simulink model "IM_Control_Sim_Current_Flux"  (R2024b)
settings: Solver=VariableStepAuto  StartTime=0.0  StopTime=200  RelTol=1e-3
InitFcn:
  | IM_parameters_init;
undefined symbols (not defined in the file): ctrl, im, Lm, Lr, Ls, p, Rr
libraries: simulink x2
settings Model: Creator=matth  LastModifiedBy=overflow

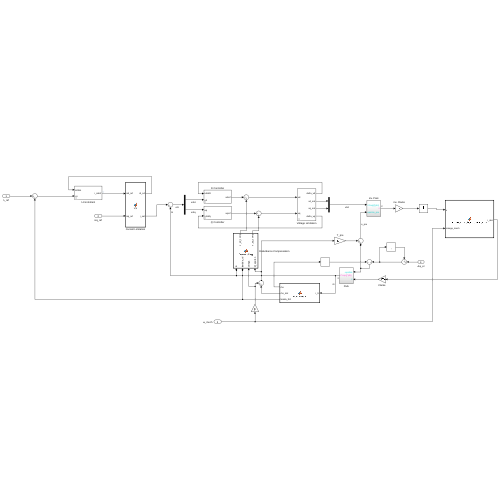
[thumbnail: Simulink's stored preview of the top-level diagram]
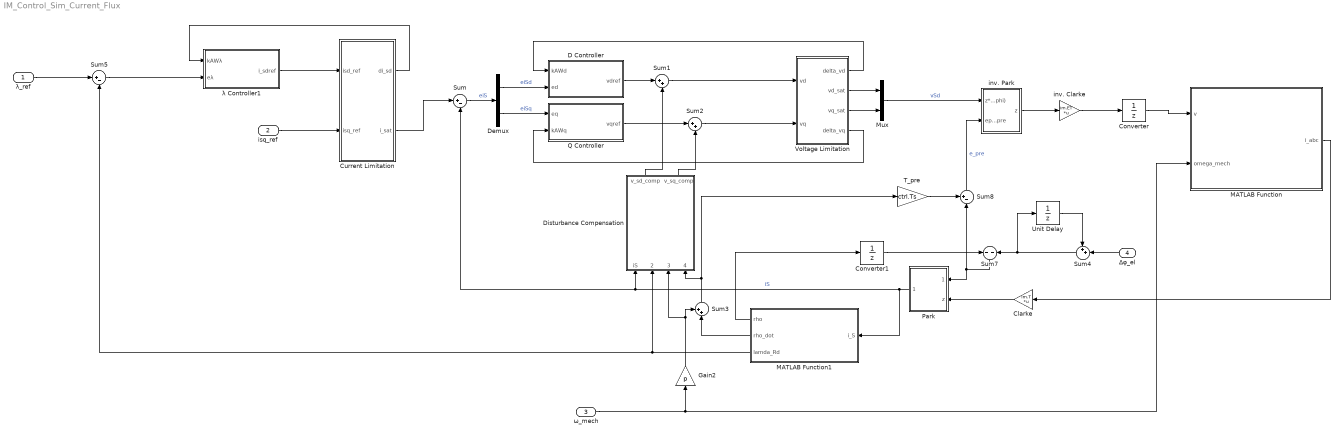
== system IM_Control_Sim_Current_Flux ==
  λ_ref : Inport
  isq_ref : Inport  Port=2
  ω_mech : Inport  Port=3
  Δφ_el : Inport  Port=4
  Clarke : Gain  Gain=im.T  Multiplication=Matrix(K*u)
  Converter : UnitDelay  SampleTime=-1  HasFrameUpgradeWarning=on
  Converter1 : UnitDelay  SampleTime=-1  HasFrameUpgradeWarning=on
  Current Limitation : MATLAB Function  TreatAsAtomicUnit=on
  D Controller : Subsystem  mask{Ts=ctrl.Ts, ctrl=ctrl.i}
      mask prompts: Ts "Sampling Time"; ctrl "Controller Struct"
  Demux : Demux  Outputs=2
  Disturbance Compensation : MATLAB Function  TreatAsAtomicUnit=on
  Gain2 : Gain  Gain=p
  MATLAB Function : MATLAB Function  TreatAsAtomicUnit=on
  MATLAB Function1 : MATLAB Function  TreatAsAtomicUnit=on
  Mux : Mux  Inputs=2
  Park : Subsystem
  Q Controller : Subsystem  mask{Ts=ctrl.Ts, ctrl=ctrl.i}
      mask prompts: Ts "Sampling Time"; ctrl "Controller Struct"
  Sum : Sum  Inputs=|+-
  Sum1 : Sum  Inputs=|++  OutDataTypeStr=double  AccumDataTypeStr=double
  Sum2 : Sum  Inputs=|++  OutDataTypeStr=double  AccumDataTypeStr=double
  Sum3 : Sum  Inputs=++|
  Sum4 : Sum  Inputs=++|
  Sum5 : Sum  Inputs=|+-
  Sum7 : Sum  Inputs=-|-
  Sum8 : Sum  Inputs=+-|
  T_pre : Gain  Gain=ctrl.Ts  SaturateOnIntegerOverflow=on  OutDataTypeStr=Inherit: Same as input  ParamDataTypeStr=Inherit: Same as input
  Unit Delay : UnitDelay  SampleTime=-1  HasFrameUpgradeWarning=on
  Voltage Limitation : Subsystem  mask{Vmax=im.vDC}
      mask prompts: Vmax "Max Voltage"
  inv. Clarke : Gain  Gain=im.ET  Multiplication=Matrix(K*u)
  inv. Park : Subsystem
  λ Controller1 : Subsystem  mask{Ts=ctrl.Ts, ctrl=ctrl.w}
      mask prompts: Ts "Sampling Time"; ctrl "Controller Struct"
  wires:
  Q Controller/1(vqref) -> Sum2/1
  Sum2/1 -> Voltage Limitation/2("vq ")
  Sum1/1 -> Voltage Limitation/1(vd)
  D Controller/1(vdref) -> Sum1/1
  Voltage Limitation/3(vq_sat) -> Mux/2
  MATLAB Function/1(i_abc) -> Clarke/1
  Mux/1 -> inv. Park/1(z*exp(j*phi))  "vSd"
  Voltage Limitation/1(delta_vd) -> D Controller/1(kAWd)
  Sum/1 -> Demux/1  "eiS"
  Demux/1 -> D Controller/2(ed)  "eiSd"
  Clarke/1 -> Park/2(z)
  inv. Park/1(z) -> inv. Clarke/1
  Demux/2 -> Q Controller/1(eq)  "eiSq"
  Park/1(z*exp(j*phi)) -> MATLAB Function1/1(i_S), Disturbance Compensation/1(iS), Sum/2  "iS"
  Voltage Limitation/4(delta_vq) -> Q Controller/2(kAWq)
  Voltage Limitation/2(vd_sat) -> Mux/1
  Converter/1 -> MATLAB Function/1(v)
  MATLAB Function1/3(lamda_Rd) -> Disturbance Compensation/2(lambda_rd), Sum5/2
  Sum3/1 -> Disturbance Compensation/4(dt_epsilon), T_pre/1
  Current Limitation/2(i_sat) -> Sum/1
  MATLAB Function1/2(rho_dot) -> Sum3/2
  Sum7/1 -> Park/1(-epsilon), Sum8/2
  T_pre/1 -> Sum8/1
  MATLAB Function1/1(rho) -> Converter1/1
  Converter1/1 -> Sum7/1
  λ Controller1/1(i_sdref) -> Current Limitation/1(isd_ref)
  Current Limitation/1(di_sd) -> λ Controller1/1(kAWλ)
  Sum5/1 -> λ Controller1/2(eλ)
  λ_ref/1 -> Sum5/1
  inv. Clarke/1 -> Converter/1
  isq_ref/1 -> Current Limitation/2(isq_ref)
  Sum8/1 -> inv. Park/2(epsilon_pre)  "e_pre"
  Disturbance Compensation/1(v_sd_comp) -> Sum1/2
  Disturbance Compensation/2(v_sq_comp) -> Sum2/2
  Gain2/1 -> Sum3/1, Disturbance Compensation/3(omega)
  ω_mech/1 -> Gain2/1, MATLAB Function/2(omega_mech)
  Δφ_el/1 -> Sum4/2
  Sum4/1 -> Unit Delay/1, Sum7/2
  Unit Delay/1 -> Sum4/1

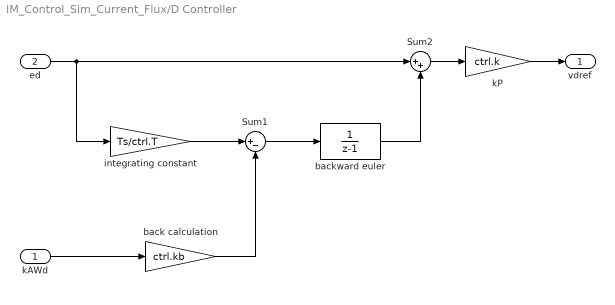
== system IM_Control_Sim_Current_Flux/D Controller ==
  kAWd : Inport
  ed : Inport  Port=2
  Sum1 : Sum  Inputs=|+-
  Sum2 : Sum  Inputs=|++
  back calculation : Gain  Gain=ctrl.kb
  backward euler : DiscreteTransferFcn  Denominator=[1 -1]
  integrating constant : Gain  Gain=Ts/ctrl.T
  kP : Gain  Gain=ctrl.k
  vdref : Outport
  wires:
  Sum1/1 -> backward euler/1
  integrating constant/1 -> Sum1/1
  back calculation/1 -> Sum1/2
  ed/1 -> integrating constant/1, Sum2/1
  Sum2/1 -> kP/1
  kP/1 -> vdref/1
  backward euler/1 -> Sum2/2
  kAWd/1 -> back calculation/1

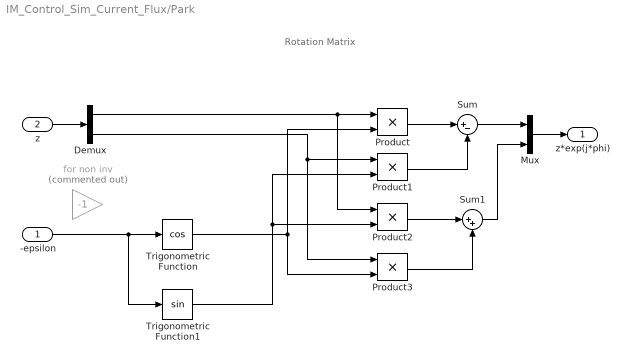
== system IM_Control_Sim_Current_Flux/Park ==
  note: Rotation Matrix
  -epsilon : Inport
  z : Inport  Port=2
  Demux : Demux  Outputs=2
      settings: DisplayOption=none
  Mux : Mux  Inputs=2
  Product{,1..3} (4 alike) : Product  SaturateOnIntegerOverflow=on  OutDataTypeStr=Inherit: Same as first input
  Sum : Sum  Inputs=|+-  SaturateOnIntegerOverflow=on
  Sum1 : Sum  Inputs=|++  SaturateOnIntegerOverflow=on
  Trigonometric Function : Trigonometry  Operator=cos
  Trigonometric Function1 : Trigonometry
  for non inv : Gain  Commented=on  Gain=-1
  z*exp(j*phi) : Outport  PortDimensions=2  VectorParamsAs1DForOutWhenUnconnected=off
  wires:
  Mux/1 -> z*exp(j*phi)/1
  Sum1/1 -> Mux/2
  Sum/1 -> Mux/1
  Product3/1 -> Sum1/2
  Product2/1 -> Sum1/1
  Product1/1 -> Sum/2
  Product/1 -> Sum/1
  Trigonometric Function1/1 -> Product2/2, Product1/2
  Trigonometric Function/1 -> Product3/2, Product/2
  Demux/2 -> Product3/1, Product1/1
  Demux/1 -> Product2/1, Product/1
  z/1 -> Demux/1
  -epsilon/1 -> Trigonometric Function1/1, Trigonometric Function/1

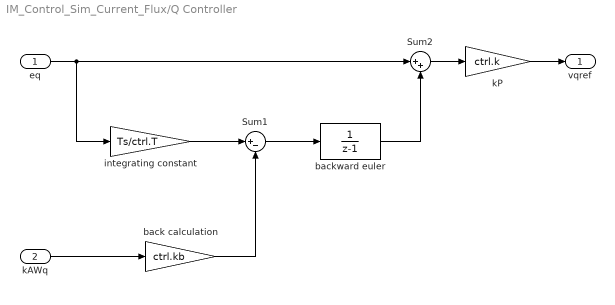
== system IM_Control_Sim_Current_Flux/Q Controller ==
  eq : Inport
  kAWq : Inport  Port=2
  Sum1 : Sum  Inputs=|+-
  Sum2 : Sum  Inputs=|++
  back calculation : Gain  Gain=ctrl.kb
  backward euler : DiscreteTransferFcn  Denominator=[1 -1]
  integrating constant : Gain  Gain=Ts/ctrl.T
  kP : Gain  Gain=ctrl.k
  vqref : Outport
  wires:
  Sum1/1 -> backward euler/1
  integrating constant/1 -> Sum1/1
  back calculation/1 -> Sum1/2
  eq/1 -> integrating constant/1, Sum2/1
  Sum2/1 -> kP/1
  kP/1 -> vqref/1
  backward euler/1 -> Sum2/2
  kAWq/1 -> back calculation/1

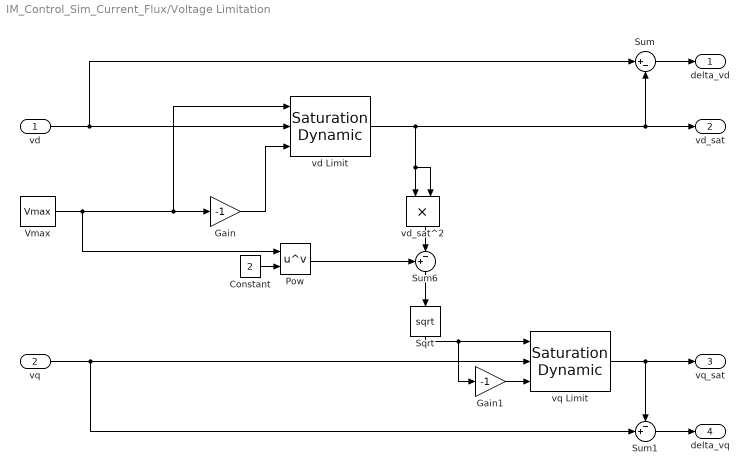
== system IM_Control_Sim_Current_Flux/Voltage Limitation ==
  vd : Inport
  "vq " : Inport  Port=2
  Constant : Constant  Value=2
  Gain : Gain  Gain=-1
  Gain1 : Gain  Gain=-1
  Pow : Math  Operator=pow  RndMeth=Zero
  Sqrt : Sqrt
  Sum : Sum  Inputs=|+-
  Sum1 : Sum  Inputs=-+|
  Sum6 : Sum  Inputs=+-|
  Vmax : Constant  Value=Vmax
  vd Limit : simulink/Discontinuities/Saturation Dynamic  OutMin=[]  OutMax=[]  OutDataTypeStr=Inherit: Same as second input  OutDataType=fixdt(1, 16)  OutScaling=2^-10  DoSatur=off
  vd_sat^2 : Product
  vq Limit : simulink/Discontinuities/Saturation Dynamic  OutMin=[]  OutMax=[]  OutDataTypeStr=Inherit: Same as second input  OutDataType=fixdt(1, 16)  OutScaling=2^-10  DoSatur=off
  delta_vd : Outport  VectorParamsAs1DForOutWhenUnconnected=off
  vd_sat : Outport  Port=2  VectorParamsAs1DForOutWhenUnconnected=off
  vq_sat : Outport  Port=3  VectorParamsAs1DForOutWhenUnconnected=off
  delta_vq : Outport  Port=4  VectorParamsAs1DForOutWhenUnconnected=off
  wires:
  Gain/1 -> vd Limit/3
  vd Limit/1 -> Sum/2, vd_sat/1, vd_sat^2/2, vd_sat^2/1
  Sqrt/1 -> Gain1/1, vq Limit/1
  vq Limit/1 -> Sum1/1, vq_sat/1
  Pow/1 -> Sum6/1
  vd/1 -> Sum/1, vd Limit/2
  Sum6/1 -> Sqrt/1
  "vq "/1 -> vq Limit/2, Sum1/2
  vd_sat^2/1 -> Sum6/2
  Vmax/1 -> Pow/1, Gain/1, vd Limit/1
  Gain1/1 -> vq Limit/3
  Sum/1 -> delta_vd/1
  Sum1/1 -> delta_vq/1
  Constant/1 -> Pow/2

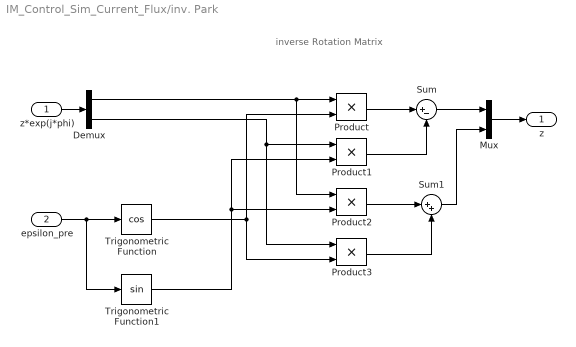
== system IM_Control_Sim_Current_Flux/inv. Park ==
  note: inverse Rotation Matrix
  z*exp(j*phi) : Inport
  epsilon_pre : Inport  Port=2
  Demux : Demux  Outputs=2
      settings: DisplayOption=none
  Mux : Mux  Inputs=2
  Product{,1..3} (4 alike) : Product  SaturateOnIntegerOverflow=on  OutDataTypeStr=Inherit: Same as first input
  Sum : Sum  Inputs=|+-  SaturateOnIntegerOverflow=on
  Sum1 : Sum  Inputs=|++  SaturateOnIntegerOverflow=on
  Trigonometric Function : Trigonometry  Operator=cos
  Trigonometric Function1 : Trigonometry
  z : Outport  PortDimensions=2  VectorParamsAs1DForOutWhenUnconnected=off
  wires:
  z*exp(j*phi)/1 -> Demux/1
  Demux/1 -> Product/1, Product2/1
  epsilon_pre/1 -> Trigonometric Function1/1, Trigonometric Function/1
  Demux/2 -> Product1/1, Product3/1
  Trigonometric Function/1 -> Product/2, Product3/2
  Trigonometric Function1/1 -> Product1/2, Product2/2
  Product/1 -> Sum/1
  Product1/1 -> Sum/2
  Product2/1 -> Sum1/1
  Product3/1 -> Sum1/2
  Sum/1 -> Mux/1
  Sum1/1 -> Mux/2
  Mux/1 -> z/1

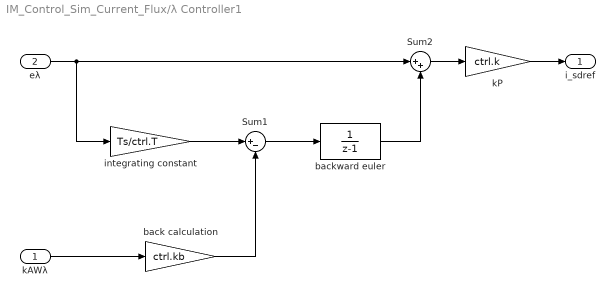
== system IM_Control_Sim_Current_Flux/λ Controller1 ==
  kAWλ : Inport
  eλ : Inport  Port=2
  Sum1 : Sum  Inputs=|+-
  Sum2 : Sum  Inputs=|++
  back calculation : Gain  Gain=ctrl.kb
  backward euler : DiscreteTransferFcn  Denominator=[1 -1]
  integrating constant : Gain  Gain=Ts/ctrl.T
  kP : Gain  Gain=ctrl.k
  i_sdref : Outport
  wires:
  Sum1/1 -> backward euler/1
  integrating constant/1 -> Sum1/1
  back calculation/1 -> Sum1/2
  eλ/1 -> integrating constant/1, Sum2/1
  Sum2/1 -> kP/1
  kP/1 -> i_sdref/1
  backward euler/1 -> Sum2/2
  kAWλ/1 -> back calculation/1

== matlab function IM_Control_Sim_Current_Flux/MATLAB Function1 ==
  data: rho output; rho_dot output; i_S input; lamda_Rd output; par parameter
function [rho, rho_dot, lamda_Rd] = flux_model(i_S, par)

i_sd = i_S(1);
i_sq = i_S(2);

% PARAMETERS
Ts = par.Ts;
p  = par.p;
Jm = par.J;

Rs = par.Rs;
Rr = par.Rr;

Ls = par.Ls;     % LσS
Lr = par.Lr;     % L'σR
Lm  = par.Lm;

Tau_R = Lr/Rr;

persistent rho_k lamda_Rd_k
if isempty(rho_k)
    rho_k = 0;
    lamda_Rd_k = 0.001;
end


lamda_Rd_k = lamda_Rd_k + Ts / Tau_R * (Lm * i_sd - lamda_Rd_k);

lamda_Rd_k = max(lamda_Rd_k, 0.001);


rho_dot = Lm * i_sq / (Tau_R * lamda_Rd_k);

rho_k = rho_k + Ts * rho_dot;

lamda_Rd = lamda_Rd_k;
rho = rho_k;

== matlab function IM_Control_Sim_Current_Flux/Disturbance Compensation ==
  data: iS input; v_sd_comp output; lambda_rd input; omega input; dt_epsilon input; Ls parameter; Lm parameter; Lr parameter; Rr parameter; v_sq_comp output
function [v_sd_comp, v_sq_comp]  = Decoupling(iS, lambda_rd, omega, dt_epsilon, Ls, Lm, Lr, Rr)

i_Sd = iS(1);
i_Sq = iS(2);

% convenience;  (3.15) unter satz
L_sigma=(Ls - Lm^2/Lr); 

% compensation
v_sd_comp = -dt_epsilon*L_sigma*i_Sq - Rr *  Lm/Lr^2 * lambda_rd;  % (3.21)
v_sq_comp =  dt_epsilon*L_sigma*i_Sd + omega * Lm/Lr^2 * lambda_rd; % (3.22)

== matlab function IM_Control_Sim_Current_Flux/MATLAB Function ==
  data: i_abc output; v input; par parameter; omega_mech input
function i_abc  = IM_mech_subsystem_vector(v,par, omega_mech)

va = v(1);
vb = v(2);
vc = v(3);

% PARAMETERS
Ts = par.Ts;
p  = par.p;

Rs = par.Rs;
Rr = par.Rr;

Ls = par.Ls;     
Lr = par.Lr;     
Lm  = par.Lm;


% Persistent states
persistent is_a is_b psir_a psir_b
if isempty(is_a)
    is_a = 0; is_b = 0;
    psir_a = 0; psir_b = 0;
end

% Clarke transform (abc -> alpha-beta), power-invariant
v_alpha = (2/3)*(va - 0.5*vb - 0.5*vc);
v_beta  = (2/3)*((sqrt(3)/2)*(vb - vc));

% Helpful constants
Lsigma = Ls - (Lm^2)/Lr;        % must be > 0
omega_r = p * omega_mech;

% Current and rotor flux vectors
is  = [is_a;  is_b];
psir = [psir_a; psir_b];

Jmat = [0 -1; 1 0];

% Rotor flux derivative: dpsir/dt
dpsir = -(Rr/Lr)*psir + (Rr*Lm/Lr)*is + omega_r*(Jmat*psir);

% Stator current derivative: dis/dt
vs = [v_alpha; v_beta];
dis = (1/Lsigma) * (vs - Rs*is - (Lm/Lr)*dpsir);

% Integrate (Euler)
psir = psir + Ts*dpsir;
is   = is   + Ts*dis;


% Save states back
is_a = is(1); is_b = is(2);
psir_a = psir(1); psir_b = psir(2);


% Inverse Clarke: alpha-beta -> abc currents (with ia+ib+ic=0)
i_a = is(1);
i_b = -0.5*is(1) + (sqrt(3)/2)*is(2);
i_c = -0.5*is(1) - (sqrt(3)/2)*is(2);

i_abc = [i_a; i_b; i_c];

end

== matlab function IM_Control_Sim_Current_Flux/Current Limitation ==
  data: isd_ref input; di_sd output; isq_ref input; i_sat output; par parameter
function [di_sd, i_sat] = fcn(isd_ref, isq_ref, par)

isd_max = par.k_is * par.is_max;

isd_sat = max([min(isd_ref, isd_max), -isd_max]);

di_sd = isd_ref - isd_sat;

isq_max = sqrt(par.is_max^2 -  isd_sat^2);

isq_sat = max([min(isq_ref, isq_max), -isq_max]);

i_sat = [isd_sat, isq_sat];
